simulink model "Demo1_L2P1A4"  (R2023a)
settings: Solver=VariableStepAuto  StartTime=0.0  StopTime=5  RelTol=1e-3
settings Model: Creator=rqouta  LastModifiedBy=rqouta

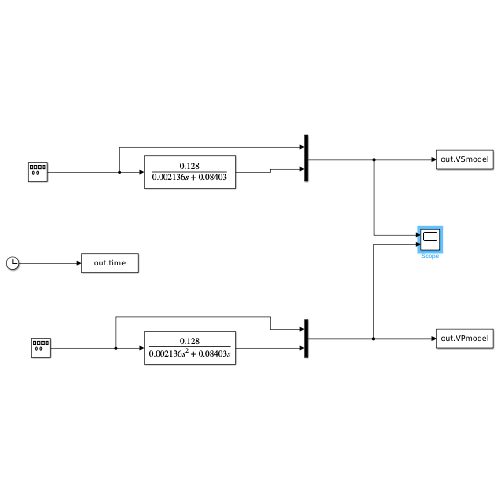
[thumbnail: Simulink's stored preview of the top-level diagram]
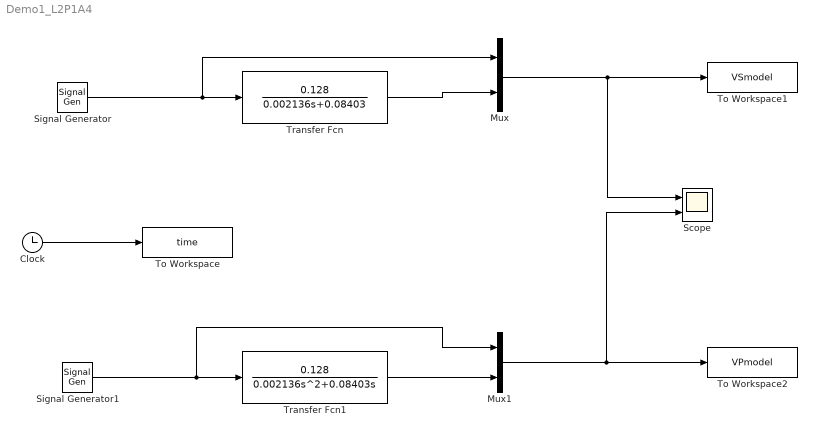
== system Demo1_L2P1A4 ==
  Clock : Clock
  Mux : Mux  Inputs=2
  Mux1 : Mux  Inputs=2
  Scope : Scope  NumInputPorts=2
  Signal Generator : SignalGenerator  WaveForm=square  Frequency=0.5
  Signal Generator1 : SignalGenerator  WaveForm=square  Frequency=0.5
  To Workspace : ToWorkspace  VariableName=time  SampleTime=-1
  To Workspace1 : ToWorkspace  VariableName=VSmodel  SampleTime=-1
  To Workspace2 : ToWorkspace  VariableName=VPmodel  SampleTime=-1
  Transfer Fcn : TransferFcn  Numerator=[0.128]  Denominator=[0.002136 0.08403]
  Transfer Fcn1 : TransferFcn  Numerator=[0.128]  Denominator=[0.002136 0.08403 0]
  wires:
  Mux1/1 -> Scope/2, To Workspace2/1
  Signal Generator1/1 -> Mux1/1, Transfer Fcn1/1
  Transfer Fcn/1 -> Mux/2
  Signal Generator/1 -> Mux/1, Transfer Fcn/1
  Mux/1 -> Scope/1, To Workspace1/1
  Clock/1 -> To Workspace/1
  Transfer Fcn1/1 -> Mux1/2
